simulink model "pendule_inverse"  (R2023a)
settings: Solver=ode1  StartTime=0.0  StopTime=10.0  RelTol=1e-3
undefined symbols (not defined in the file): K, ue, xe
settings Model: Creator=fhudrisi  LastModifiedBy=mra4306
settings OptimizationCC: ReuseModelBlockBuffer=off
settings DebuggingCC: AlgebraicLoopMsg=none  UnconnectedInputMsg=warning  UnconnectedOutputMsg=warning  UnconnectedLineMsg=warning
settings ModelReferenceCC: EnableRefExpFcnMdlSchedulingChecks=on
settings RTWCC: DLArmComputeVersion=19.05

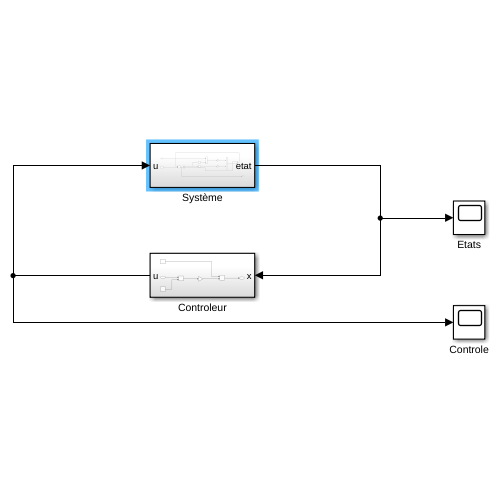
[thumbnail: Simulink's stored preview of the top-level diagram]
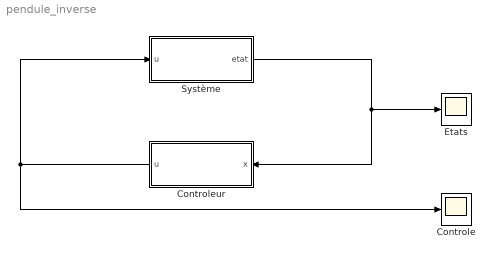
== system pendule_inverse ==
  Controle : Scope
  Controleur : Subsystem
  Etats : Scope
  Système : Subsystem
  wires:
  Controleur/1(u) -> Système/1(u), Controle/1
  Système/1(etat) -> Controleur/1(x), Etats/1

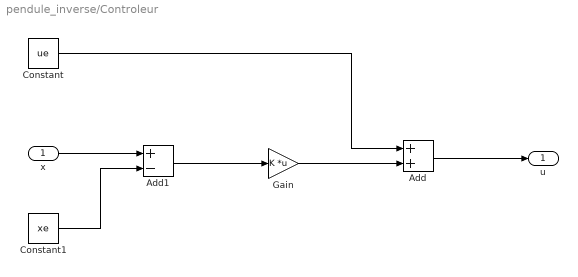
== system pendule_inverse/Controleur ==
  x : Inport
  Add : Sum
  Add1 : Sum  Inputs=+-
  Constant : Constant  Value=ue
  Constant1 : Constant  Value=xe
  Gain : Gain  Gain=K  Multiplication=Matrix(K*u)
  u : Outport
  wires:
  x/1 -> Add1/1
  Constant1/1 -> Add1/2
  Add1/1 -> Gain/1
  Constant/1 -> Add/1
  Gain/1 -> Add/2
  Add/1 -> u/1

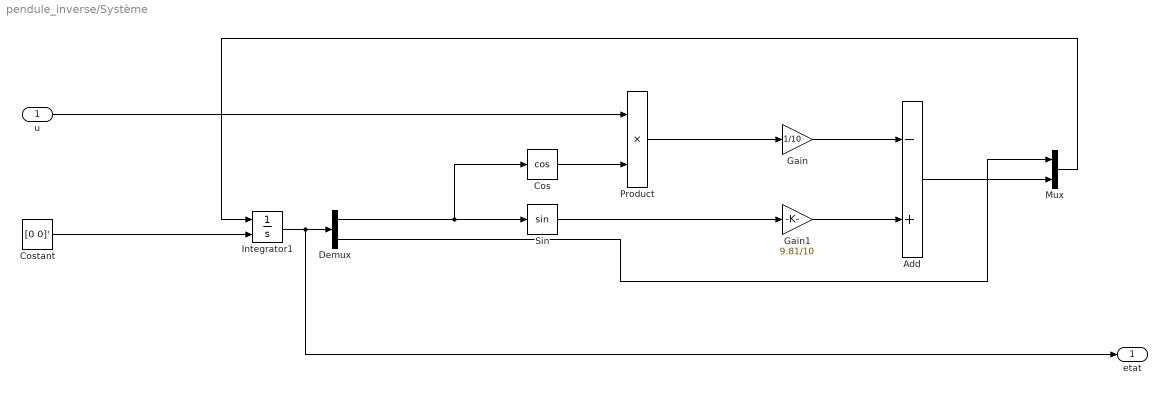
== system pendule_inverse/Système ==
  u : Inport
  Add : Sum  Inputs=-+
  Cos : Trigonometry  Operator=cos
  Costant : Constant  Value=[0 0]'
  Demux : Demux  Outputs=2
  Gain : Gain  Gain=1/10
  Gain1 : Gain  Gain=9.81/10
  Integrator1 : Integrator  InitialConditionSource=external
  Mux : Mux  Inputs=2
  Product : Product
  Sin : Trigonometry
  etat : Outport
  wires:
  Costant/1 -> Integrator1/2
  Integrator1/1 -> etat/1, Demux/1
  Demux/1 -> Sin/1, Cos/1
  Cos/1 -> Product/2
  u/1 -> Product/1
  Product/1 -> Gain/1
  Gain/1 -> Add/1
  Sin/1 -> Gain1/1
  Gain1/1 -> Add/2
  Add/1 -> Mux/2
  Demux/2 -> Mux/1
  Mux/1 -> Integrator1/1
